simulink subsystem "Orbit"  (R2021b)
settings: Solver=VariableStepAuto  StartTime=0.0  StopTime=10.0  RelTol=1e-3
undefined symbols (not defined in the file): Earth, WGS84
libraries: mbdriLib x5, aerolibtransform2 x1
settings Model: Creator=promero  LastModifiedBy=promero

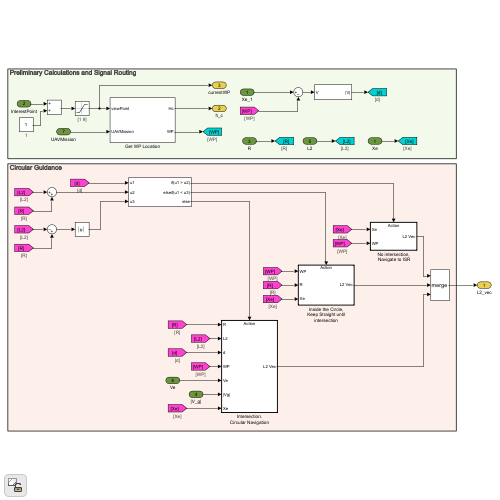
[thumbnail: Simulink's stored preview of the top-level diagram]
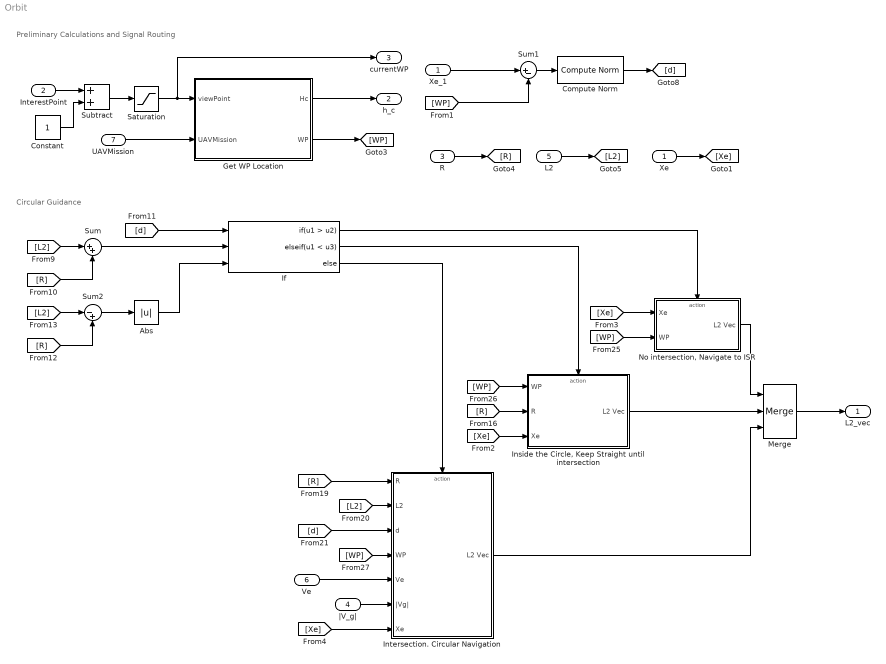
== system Orbit ==
  note: Preliminary Calculations and Signal Routing
  note: Circular Guidance
  Xe : Inport  RequirementInfo={} %GIDa_2e925e0f_56fd_456e_aab0_3db3991cd8a5
  InterestPoint : Inport  RequirementInfo={} %GIDa_3bca4efe_25ab_4f1c_b2eb_090cde379173  Port=2
  R : Inport  RequirementInfo={} %GIDa_ac40e73e_1440_4447_a901_fdaa9463ba50  Port=3
  |V_g| : Inport  RequirementInfo={} %GIDa_8e96ecb3_1b01_4fe1_9209_78720fbb68e6  Port=4
  L2 : Inport  RequirementInfo={} %GIDa_ab27639b_9d46_4779_ba6f_619c92fbb682  Port=5
  Ve : Inport  RequirementInfo={} %GIDa_a2923614_a95f_44f3_9b97_f5d4d2370fbf  Port=6
  UAVMission : Inport  RequirementInfo={} %GIDa_2e0a40cc_111d_4da8_9ca0_e3007c0c9f42  Port=7
  " Compute Norm" : mbdriLib/Utilities/ Compute Norm  SystemSampleTime=-1  VariantActivationTime=update diagram  Latency=0  AutoFrameSizeCalculation=off
  Abs : Abs  RequirementInfo={} %GIDa_97a92e8f_9fe4_4ab2_96d6_c5f0648eea8a
  Constant : Constant  RequirementInfo={} %GIDa_973cce71_8a2d_4574_843d_a33d14755dc9  OutDataTypeStr=uint8
      settings: AttributesFormatString=%<Value>
  Get WP Location : Subsystem  RequirementInfo={} %GIDa_94e8a342_81cd_4ea9_a56e_dd5849e58f84
  If : If  RequirementInfo={} %GIDa_bfc453c8_5d8c_46b5_9509_12167fc0f011  NumInputs=3  IfExpression=u1 > u2  ElseIfExpressions=u1 < u3
  "Inside the Circle, Keep Straight until intersection" : Subsystem  RequirementInfo={} %GIDa_ab8d9ba8_5a25_47f9_8f06_a28c4f1f2758  TreatAsAtomicUnit=on
  Intersection. Circular Navigation : Subsystem  RequirementInfo={} %GIDa_56d45a2c_5275_4f5d_99db_331d04595cf6  TreatAsAtomicUnit=on
  Merge : Merge  RequirementInfo={} %GIDa_e44fdab2_c75e_4c4a_a4c2_45dddf4c0c88  Inputs=3
  "No intersection, Navigate to ISR" : Subsystem  RequirementInfo={} %GIDa_d0dd1591_de8e_447f_b810_d45337d34323  TreatAsAtomicUnit=on
  Saturation : Saturate  RequirementInfo={} %GIDa_b2957e06_194f_49a6_8b1c_f700b6306751  UpperLimit=9  LowerLimit=1
      settings: AttributesFormatString=[%<LowerLimit> %<UpperLimit>]
  Subtract : Sum  RequirementInfo={} %GIDa_d5379667_99ee_4386_9924_336d8af93e7f  Inputs=2
  Sum : Sum  RequirementInfo={} %GIDa_0168e284_2b07_4503_a998_962f3a3bf7c2  Inputs=|++
  Sum1 : Sum  RequirementInfo={} %GIDa_121a286e_bee0_4533_8169_fbdc6bd0e2a0  Inputs=|+-
  Sum2 : Sum  RequirementInfo={} %GIDa_820d94db_e0e8_467a_8e6a_1a977b572eaf  Inputs=|-+
  Xe_1 : InportShadow  RequirementInfo={} %GIDa_e04ed7ee_6372_462d_bb41_1657b8eb89da
  L2_vec : Outport  RequirementInfo={} %GIDa_314a0a37_d45d_4761_aa83_cad5a0ae48ec  VectorParamsAs1DForOutWhenUnconnected=off
  h_c : Outport  RequirementInfo={} %GIDa_d111f4d9_8fff_4790_8546_4ad7a16acde2  Port=2  VectorParamsAs1DForOutWhenUnconnected=off
  currentWP : Outport  RequirementInfo={} %GIDa_256dce93_5f97_4d0a_85ba_8432794be03b  Port=3  VectorParamsAs1DForOutWhenUnconnected=off
  wires:
  R/1 -> [R]
  [Xe] -> "No intersection, Navigate to ISR"/1(Xe)
  Subtract/1 -> Saturation/1
  Constant/1 -> Subtract/2
  [Xe] -> "Inside the Circle, Keep Straight until intersection"/3(Xe)
  L2/1 -> [L2]
  Intersection. Circular Navigation/1(L2 Vec) -> Merge/3
  Xe/1 -> [Xe]
  InterestPoint/1 -> Subtract/1
  [R] -> Intersection. Circular Navigation/1(R)
  "Inside the Circle, Keep Straight until intersection"/1(L2 Vec) -> Merge/2
  "No intersection, Navigate to ISR"/1(L2 Vec) -> Merge/1
  Sum/1 -> If/2
  " Compute Norm"/1 -> [d]
  [R] -> Sum/2
  Sum1/1 -> " Compute Norm"/1
  Get WP Location/1(Hc) -> h_c/1
  UAVMission/1 -> Get WP Location/2(UAVMission)
  Get WP Location/2(WP) -> [WP]
  [R] -> "Inside the Circle, Keep Straight until intersection"/2(R)
  [WP] -> Intersection. Circular Navigation/4(WP)
  [R] -> Sum2/2
  If/2 -> "Inside the Circle, Keep Straight until intersection"/Action
  Sum2/1 -> Abs/1
  [WP] -> "Inside the Circle, Keep Straight until intersection"/1(WP)
  Merge/1 -> L2_vec/1
  [L2] -> Sum2/1
  Abs/1 -> If/3
  |V_g|/1 -> Intersection. Circular Navigation/6(|Vg|)
  [WP] -> "No intersection, Navigate to ISR"/2(WP)
  Xe_1/1 -> Sum1/1
  [WP] -> Sum1/2
  [d] -> If/1
  Ve/1 -> Intersection. Circular Navigation/5(Ve)
  [d] -> Intersection. Circular Navigation/3(d)
  If/1 -> "No intersection, Navigate to ISR"/Action
  If/3 -> Intersection. Circular Navigation/Action
  [L2] -> Sum/1
  Saturation/1 -> Get WP Location/1(viewPoint), currentWP/1
  [L2] -> Intersection. Circular Navigation/2(L2)
  [Xe] -> Intersection. Circular Navigation/7(Xe)

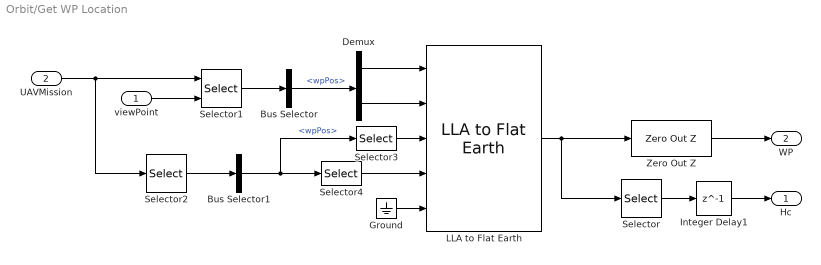
== system Orbit/Get WP Location ==
  viewPoint : Inport  RequirementInfo={} %GIDa_6a53143b_ba04_4d0a_8010_6135e561d307
  UAVMission : Inport  RequirementInfo={} %GIDa_c081361f_0229_491e_81ae_bd103e863b5b  Port=2
  Bus Selector : BusSelector  RequirementInfo={} %GIDa_01ab0b3b_b211_4260_b411_62c209cf347d  OutputSignals=wpPos
  Bus Selector1 : BusSelector  RequirementInfo={} %GIDa_87d5590e_01ce_4445_970c_d3d4a427b52e  OutputSignals=wpPos
  Demux : Demux  RequirementInfo={} %GIDa_242922ac_b249_4314_8aa6_e805d4b64783  Outputs=[2 1]
  Ground : Ground  RequirementInfo={} %GIDa_804df71d_2482_4797_934e_261bec587815
  Integer Delay1 : Delay  RequirementInfo={} %GIDa_d79a877d_60d7_4d45_bd6c_79062b758d5f  DelayLength=1
  LLA to Flat Earth : aerolibtransform2/LLA to Flat Earth  RequirementInfo={} %GIDa_da2a5ca5_2a6c_4f71_ae7c_e1af79aa7b7f  units=Metric (MKS)  ptype=Earth (WGS84)  F=1/298.257223563  R=6378137  refPosPort=on  LL0=[0 10]  psi=0
      settings: SourceProductBaseCode=AE
  Selector : Selector  RequirementInfo={} %GIDa_c26275bc_b023_446e_b08f_cef804abcb54  InputPortWidth=3  IndexOptions=Index vector (dialog)  Indices=[3]  OutputSizes=1
  Selector1 : Selector  RequirementInfo={} %GIDa_8ea0fd9a_c438_46a9_8d0b_707d7048a188  InputPortWidth=10  IndexOptions=Index vector (port)  Indices=[3]  OutputSizes=1
  Selector2 : Selector  RequirementInfo={} %GIDa_85cff84a_9077_4e7a_b9ae_bd4075c7d976  InputPortWidth=10  IndexOptions=Index vector (dialog)  Indices=[1]  OutputSizes=1
  Selector3 : Selector  RequirementInfo={} %GIDa_166deec1_35d7_473b_bada_5d884c4b34e8  InputPortWidth=3  IndexOptions=Index vector (dialog)  Indices=[3]  OutputSizes=1
  Selector4 : Selector  RequirementInfo={} %GIDa_0eabb78f_6367_48b8_9014_6931deae0f35  InputPortWidth=3  IndexOptions=Index vector (dialog)  Indices=[1 2]  OutputSizes=1
  Zero Out Z : mbdriLib/Utilities/Zero Out Z  RequirementInfo={} %GIDa_7ab51636_a299_46f1_9e8a_ccfb06b06651  SystemSampleTime=-1  VariantActivationTime=update diagram  Latency=0  AutoFrameSizeCalculation=off
  Hc : Outport  RequirementInfo={} %GIDa_66e9a083_33e4_4e37_9ac2_e31138d5f1d2  VectorParamsAs1DForOutWhenUnconnected=off
  WP : Outport  RequirementInfo={} %GIDa_4bb6da41_2565_45d6_bec1_600583fc7ac0  Port=2  VectorParamsAs1DForOutWhenUnconnected=off
  wires:
  Ground/1 -> LLA to Flat Earth/5
  Bus Selector1/1 -> Selector3/1, Selector4/1  "<wpPos>"
  Selector/1 -> Integer Delay1/1
  Integer Delay1/1 -> Hc/1
  UAVMission/1 -> Selector2/1, Selector1/1
  viewPoint/1 -> Selector1/2
  Selector1/1 -> Bus Selector/1
  Bus Selector/1 -> Demux/1  "<wpPos>"
  Demux/2 -> LLA to Flat Earth/2
  Demux/1 -> LLA to Flat Earth/1
  Selector3/1 -> LLA to Flat Earth/3
  Selector2/1 -> Bus Selector1/1
  Selector4/1 -> LLA to Flat Earth/4
  LLA to Flat Earth/1 -> Selector/1, Zero Out Z/1
  Zero Out Z/1 -> WP/1

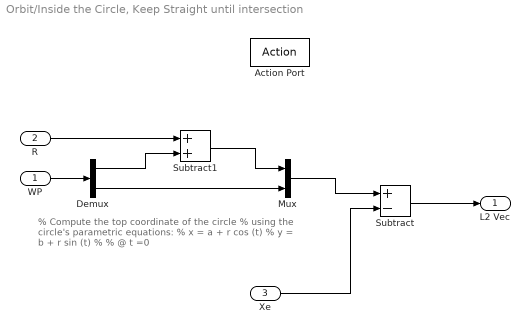
== system Orbit/Inside the Circle, Keep Straight until intersection ==
  note: % Compute the top coordinate of the circle
      | % using the circle's parametric equations:
      | % x = a + r cos (t)
      | % y = b + r sin (t)
      | %
      | % @ t =0
  WP : Inport  RequirementInfo={} %GIDa_54f4de15_201d_463e_8fdd_34b0ebfa616a
  R : Inport  RequirementInfo={} %GIDa_cac7358c_8664_42ca_a7ba_b6f04f3de72b  Port=2
  Xe : Inport  RequirementInfo={} %GIDa_6b33482a_781d_419c_9b3a_5b60b8f59437  Port=3
  Action Port : ActionPort  RequirementInfo={} %GIDa_be02cbb0_e16d_4928_8ad9_d18881738c55
  Demux : Demux  RequirementInfo={} %GIDa_8292365c_739d_4757_a2a9_ca7d36b99108  Outputs=[1 2]
  Mux : Mux  RequirementInfo={} %GIDa_b7bf9693_5d1b_490e_9003_065b0a0048f7  Inputs=2
  Subtract : Sum  RequirementInfo={} %GIDa_c8836b62_f133_4040_b82a_39e3f2045100  Inputs=+-
  Subtract1 : Sum  RequirementInfo={} %GIDa_82e7999d_8274_4aff_a953_3eb97d8c4e7a
  L2 Vec : Outport  RequirementInfo={} %GIDa_be1f331c_15e9_441d_880a_b30b065fb1ea  VectorParamsAs1DForOutWhenUnconnected=off
  wires:
  Subtract/1 -> L2 Vec/1
  Xe/1 -> Subtract/2
  Demux/1 -> Subtract1/2
  Subtract1/1 -> Mux/1
  Demux/2 -> Mux/2
  R/1 -> Subtract1/1
  WP/1 -> Demux/1
  Mux/1 -> Subtract/1

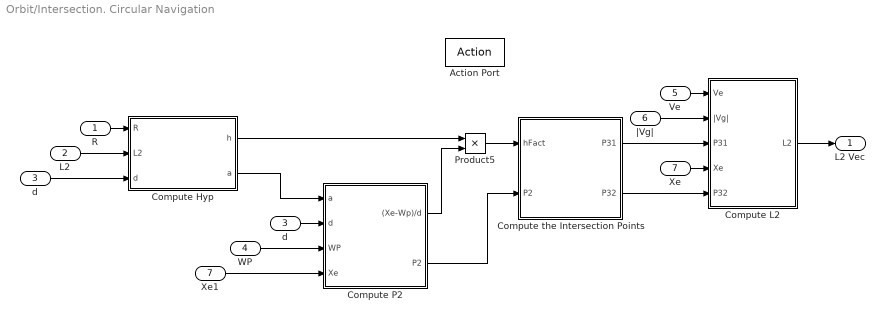
== system Orbit/Intersection. Circular Navigation ==
  R : Inport  RequirementInfo={} %GIDa_86005463_dd22_4f1d_b187_ab300998bb71
  L2 : Inport  RequirementInfo={} %GIDa_79e9c13f_1f42_4706_99fa_499263483e10  Port=2
  d : Inport  RequirementInfo={} %GIDa_39e09ba4_b0ca_4178_a03e_0e83c178e0e5  Port=3
  WP : Inport  RequirementInfo={} %GIDa_9c97f0a5_efb3_491d_bc92_0a391049b063  Port=4
  Ve : Inport  RequirementInfo={} %GIDa_7038e285_1f34_46a5_b502_5fa0889a6f54  Port=5
  |Vg| : Inport  RequirementInfo={} %GIDa_4f321b28_f958_429d_a60e_b4fb4703aca3  Port=6
  Xe : Inport  RequirementInfo={} %GIDa_c4b3f523_d779_48da_8edb_1a0a349d7a2c  Port=7
  Action Port : ActionPort  RequirementInfo={} %GIDa_efcf2185_9f0c_4a04_a783_93802d0cbd8d
  Compute Hyp : Subsystem  RequirementInfo={} %GIDa_31fce3df_e397_49b0_95be_2bca67fb115f
  Compute L2 : Subsystem  RequirementInfo={} %GIDa_4e2d04ef_25c0_4064_a338_e65bbe2a41f2
  Compute P2 : Subsystem  RequirementInfo={} %GIDa_99aa0cab_c31d_4411_88e5_8d960a8de4df
  Compute the Intersection Points : MATLAB Function  RequirementInfo={} %GIDa_454e1d20_cf0e_4112_ba75_c4eeb1ed14f9  TreatAsAtomicUnit=on
  Product5 : Product  RequirementInfo={} %GIDa_67c3cbb9_54e6_4c2a_acbc_5e7bf43e6edb  RndMeth=Zero
  Xe1 : InportShadow  RequirementInfo={} %GIDa_8eb80982_15f2_4111_a791_243f652b52c3  Port=7
  "d " : InportShadow  RequirementInfo={} %GIDa_20ac21d1_1de7_4944_b8fc_0350ab8e510e  Port=3
  L2 Vec : Outport  RequirementInfo={} %GIDa_7fd78b24_975f_42a2_a722_cfebe9dc9496  VectorParamsAs1DForOutWhenUnconnected=off
  wires:
  Product5/1 -> Compute the Intersection Points/1(hFact)
  R/1 -> Compute Hyp/1(R)
  L2/1 -> Compute Hyp/2(L2)
  d/1 -> Compute Hyp/3(d)
  Compute Hyp/1(h) -> Product5/1
  Compute Hyp/2(a) -> Compute P2/1(a)
  "d "/1 -> Compute P2/2(d)
  WP/1 -> Compute P2/3(WP)
  Xe1/1 -> Compute P2/4(Xe)
  Compute P2/1((Xe-Wp)/d) -> Product5/2
  Compute P2/2(P2) -> Compute the Intersection Points/2(P2)
  Ve/1 -> Compute L2/1(Ve)
  |Vg|/1 -> Compute L2/2(|Vg|)
  Compute the Intersection Points/1(P31) -> Compute L2/3(P31)
  Xe/1 -> Compute L2/4(Xe)
  Compute the Intersection Points/2(P32) -> Compute L2/5(P32)
  Compute L2/1(L2) -> L2 Vec/1

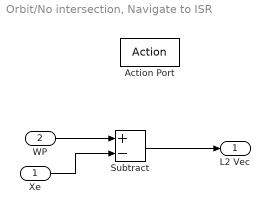
== system Orbit/No intersection, Navigate to ISR ==
  Xe : Inport  RequirementInfo={} %GIDa_c261557c_5772_4ed7_889a_746a31b114f8
  WP : Inport  RequirementInfo={} %GIDa_da23db0a_1e48_466f_adad_45602faed702  Port=2
  Action Port : ActionPort  RequirementInfo={} %GIDa_32b5d41d_a285_49a3_bb64_7d090b0300d4
  Subtract : Sum  RequirementInfo={} %GIDa_c511e9c6_eaf8_4d5a_801a_29411e6656ae  Inputs=+-
  L2 Vec : Outport  RequirementInfo={} %GIDa_9f3bdd5c_9144_43b9_894c_96b1b0d39b65  VectorParamsAs1DForOutWhenUnconnected=off
  wires:
  Subtract/1 -> L2 Vec/1
  Xe/1 -> Subtract/2
  WP/1 -> Subtract/1

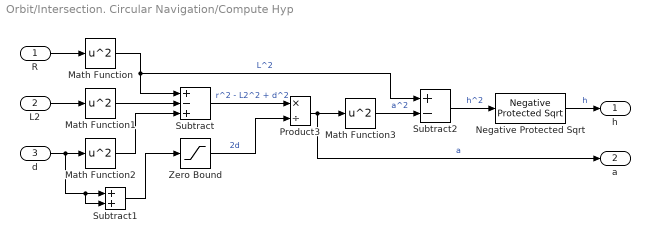
== system Orbit/Intersection. Circular Navigation/Compute Hyp ==
  R : Inport  RequirementInfo={} %GIDa_9b5da47e_6cba_4a67_a8e6_016c3d197b08
  L2 : Inport  RequirementInfo={} %GIDa_5a32c3a3_368c_4aa4_a3ae_24d84cf9473b  Port=2
  d : Inport  RequirementInfo={} %GIDa_55bb5c4b_37ee_48c5_997d_10883dc06afe  Port=3
  Math Function : Math  RequirementInfo={} %GIDa_867ad13a_2de8_424f_b1fb_b9f2648539f5  Operator=square  SignedPower=on  SaturateOnIntegerOverflow=on
  Math Function1 : Math  RequirementInfo={} %GIDa_e2557aa5_cf36_4308_8d9a_311dcd09f6f0  Operator=square  SignedPower=on  SaturateOnIntegerOverflow=on
  Math Function2 : Math  RequirementInfo={} %GIDa_f393a595_546f_4ddb_a73a_2e0399295bcd  Operator=square  SignedPower=on  SaturateOnIntegerOverflow=on
  Math Function3 : Math  RequirementInfo={} %GIDa_d6dcc4df_bd1f_4493_8c84_8199990a080f  Operator=square  SignedPower=on  SaturateOnIntegerOverflow=on
  Negative Protected Sqrt : mbdriLib/Utilities/Negative Protected Sqrt  RequirementInfo={} %GIDa_2fb03c12_f602_4e2f_ac71_f525e45e72e6  SystemSampleTime=-1  VariantActivationTime=update diagram  Latency=0  AutoFrameSizeCalculation=off
  Product3 : Product  RequirementInfo={} %GIDa_ce291192_6c2d_4680_a25b_c6704cf0389e  Inputs=*/  RndMeth=Zero
  Subtract : Sum  RequirementInfo={} %GIDa_02deb013_80c7_4484_84b8_31846bb14833  Inputs=+-+
  Subtract1 : Sum  RequirementInfo={} %GIDa_d08c68fa_d361_45e2_aa67_fd984671f965  Inputs=2
  Subtract2 : Sum  RequirementInfo={} %GIDa_4ebb57ac_e1a2_4820_9931_e1a25dd19759  Inputs=+-
  Zero Bound : Saturate  RequirementInfo={} %GIDa_b53dd1fe_4923_461a_917b_14566fde5b31  UpperLimit=inf  LowerLimit=0.001
      settings: AttributesFormatString="[%<LowerLimit>  %<UpperLimit>]"
  h : Outport  RequirementInfo={} %GIDa_dd29fa04_856f_4fc9_97fd_af773fb44016  VectorParamsAs1DForOutWhenUnconnected=off
  a : Outport  RequirementInfo={} %GIDa_f8926b0b_9704_4225_b3b4_9f40d7f8b730  Port=2  VectorParamsAs1DForOutWhenUnconnected=off
  wires:
  Math Function2/1 -> Subtract/3
  Math Function3/1 -> Subtract2/2  "a^2"
  Subtract2/1 -> Negative Protected Sqrt/1  "h^2"
  Product3/1 -> a/1, Math Function3/1  "a"
  Subtract1/1 -> Zero Bound/1
  Zero Bound/1 -> Product3/2  "2d"
  Subtract/1 -> Product3/1  "r^2 - L2^2 + d^2"
  Math Function1/1 -> Subtract/2
  Math Function/1 -> Subtract2/1, Subtract/1  "L^2"
  d/1 -> Subtract1/2, Subtract1/1, Math Function2/1
  L2/1 -> Math Function1/1
  R/1 -> Math Function/1
  Negative Protected Sqrt/1 -> h/1  "h"

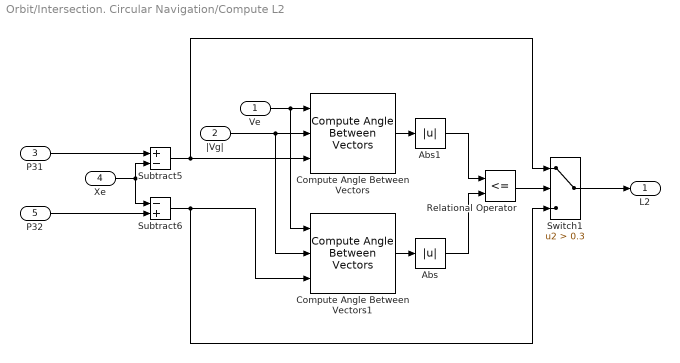
== system Orbit/Intersection. Circular Navigation/Compute L2 ==
  Ve : Inport  RequirementInfo={} %GIDa_f54482ce_0a18_4ab3_8104_b7654e2e4bbb
  |Vg| : Inport  RequirementInfo={} %GIDa_c66cdb5c_42d3_46f0_8d0f_9be45ad14bef  Port=2
  P31 : Inport  RequirementInfo={} %GIDa_b0697490_ca20_4007_9d7a_53c67ad879b0  Port=3
  Xe : Inport  RequirementInfo={} %GIDa_2156502f_d56e_45ca_9768_f676e4d3386a  Port=4
  P32 : Inport  RequirementInfo={} %GIDa_16d06e08_0773_4180_a819_866b09f6ee9b  Port=5
  Abs : Abs  RequirementInfo={} %GIDa_d3aa1c46_41a7_4697_a882_5b2288f98a15
  Abs1 : Abs  RequirementInfo={} %GIDa_feaf7071_9b26_43af_bdb5_3f2b01902ebb
  Compute Angle Between Vectors : mbdriLib/Utilities/Compute Angle Between Vectors  RequirementInfo={} %GIDa_ae33eae1_08a2_45a5_85fa_f27040195270  SystemSampleTime=-1  VariantActivationTime=update diagram  Latency=0  AutoFrameSizeCalculation=off
  Compute Angle Between Vectors1 : mbdriLib/Utilities/Compute Angle Between Vectors  RequirementInfo={} %GIDa_7309b679_c5d4_4a60_bc58_dc44e9677557  SystemSampleTime=-1  VariantActivationTime=update diagram  Latency=0  AutoFrameSizeCalculation=off
  Relational Operator : RelationalOperator  RequirementInfo={} %GIDa_8d534048_3b76_4fb9_b77c_57ad0977c7b7  Operator=<=  OutDataTypeStr=boolean  RndMeth=Nearest
  Subtract5 : Sum  RequirementInfo={} %GIDa_901ce241_dd1b_4e8b_8eef_14c009fdb60a  Inputs=+-
  Subtract6 : Sum  RequirementInfo={} %GIDa_404ace61_1d7f_47e2_8714_69c1c4bae20d  Inputs=-+
  Switch1 : Switch  RequirementInfo={} %GIDa_90c8728e_a24f_4ebb_8124_0d942c295e96  Criteria=u2 > Threshold  Threshold=0.3  ZeroCross=off
  L2 : Outport  RequirementInfo={} %GIDa_a7735d67_471e_40e4_abdf_cf2435f96294  VectorParamsAs1DForOutWhenUnconnected=off
  wires:
  Switch1/1 -> L2/1
  Xe/1 -> Subtract6/1, Subtract5/2
  P32/1 -> Subtract6/2
  Subtract6/1 -> Switch1/3, Compute Angle Between Vectors1/3
  P31/1 -> Subtract5/1
  Subtract5/1 -> Switch1/1, Compute Angle Between Vectors/3
  Relational Operator/1 -> Switch1/2
  Abs/1 -> Relational Operator/2
  Abs1/1 -> Relational Operator/1
  Compute Angle Between Vectors1/1 -> Abs/1
  Compute Angle Between Vectors/1 -> Abs1/1
  |Vg|/1 -> Compute Angle Between Vectors/2, Compute Angle Between Vectors1/2
  Ve/1 -> Compute Angle Between Vectors/1, Compute Angle Between Vectors1/1

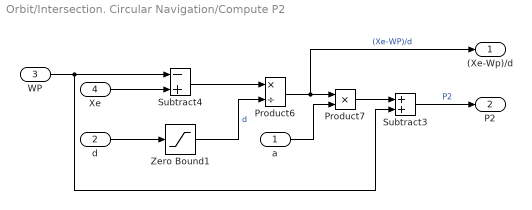
== system Orbit/Intersection. Circular Navigation/Compute P2 ==
  a : Inport  RequirementInfo={} %GIDa_0415e3d9_031a_4c69_80dd_5087414fc7a9
  d : Inport  RequirementInfo={} %GIDa_8f6b5009_d182_4e62_849c_7f7674cd0bb9  Port=2
  WP : Inport  RequirementInfo={} %GIDa_f3e226e2_42c4_4df2_acb9_b98dd7bfc4b9  Port=3
  Xe : Inport  RequirementInfo={} %GIDa_516ecfc4_1cb1_42f9_aacf_85b1e217f4e5  Port=4
  Product6 : Product  RequirementInfo={} %GIDa_dc489e9f_92a8_4072_8dbc_e349a4a26941  Inputs=*/  RndMeth=Zero
  Product7 : Product  RequirementInfo={} %GIDa_43991501_edaf_488d_8b05_e988d6f40096  RndMeth=Zero
  Subtract3 : Sum  RequirementInfo={} %GIDa_1faed134_670c_4817_a605_c06b3d54cdba  Inputs=2
  Subtract4 : Sum  RequirementInfo={} %GIDa_672515d9_f0de_411e_a776_53587491ff16  Inputs=-+
  Zero Bound1 : Saturate  RequirementInfo={} %GIDa_f4b33e9f_89d1_4db4_9a53_0d7acc0235fe  UpperLimit=inf  LowerLimit=0.001
      settings: AttributesFormatString="[%<LowerLimit>  %<UpperLimit>]"
  (Xe-Wp)/d : Outport  RequirementInfo={} %GIDa_72d88838_a444_4272_9b52_30eb9dc847cc  VectorParamsAs1DForOutWhenUnconnected=off
  P2 : Outport  RequirementInfo={} %GIDa_45219c06_0860_43ea_b2f9_4d430748011a  Port=2  VectorParamsAs1DForOutWhenUnconnected=off
  wires:
  WP/1 -> Subtract4/1, Subtract3/2
  Product7/1 -> Subtract3/1
  Xe/1 -> Subtract4/2
  Subtract4/1 -> Product6/1
  d/1 -> Zero Bound1/1
  Zero Bound1/1 -> Product6/2  "d"
  Product6/1 -> (Xe-Wp)/d/1, Product7/1  "(Xe-WP)/d"
  Subtract3/1 -> P2/1  "P2"
  a/1 -> Product7/2

== matlab function Orbit/Intersection. Circular Navigation/Compute the Intersection Points ==
  data: hFact input; P31 output; P2 input; P32 output
function [P31,P32] = getP3s(hFact, P2)
% #codegen

P31 = single([0 0 0]');
P32 = single([0 0 0]');

P31(1) = P2(1) + hFact(2);
P31(2) = P2(2) - hFact(1);

P32(1) = P2(1) - hFact(2);
P32(2) = P2(2) + hFact(1);
